simulink model "EntrySend"  (R2020b)
settings: Solver=VariableStepAuto  StartTime=0.0  StopTime=10.0  RelTol=1e-3
settings Model: Creator=apple  LastModifiedBy=apple

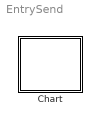
== system EntrySend ==
  Chart : Stateflow chart  TreatAsAtomicUnit=on

== stateflow chart EntrySend/Chart ==
  state A
    en:fprintf("Entry A");
    du:fprintf("During A");
    ex:fprintf("Exit A");
  state B
    en:fprintf("Entry B");send(F);
    du:fprintf("During B");
    ex:fprintf("Exit B");
  (default) -> A
  A -> B : E/{send(F);}
  B -> A : F
  events: E local FUNCTION_CALL_EVENT; F local FUNCTION_CALL_EVENT
